simulink model "task_1"  (R2024a)
settings: Solver=VariableStepAuto  StartTime=0.0  StopTime=10.0  RelTol=1e-3
libraries: simulink x1
settings Model: Creator=alexe  LastModifiedBy=alexe

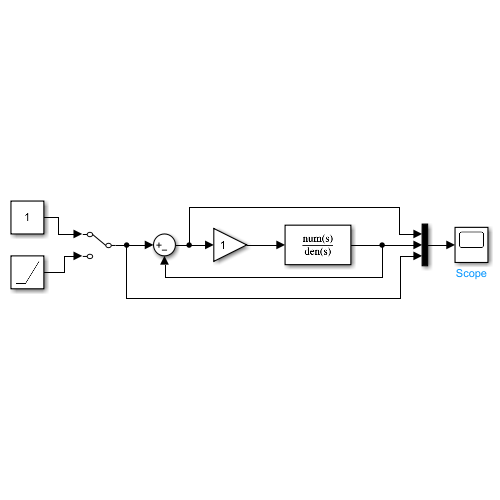
[thumbnail: Simulink's stored preview of the top-level diagram]
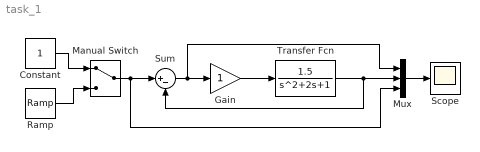
== system task_1 ==
  Constant : Constant
  Gain : Gain
  Manual Switch : ManualSwitch
  Mux : Mux  Inputs=3
  Ramp : simulink/Sources/Ramp  slope=1  start=0  InitialOutput=0
  Scope : Scope
  Sum : Sum  Inputs=|+-
  Transfer Fcn : TransferFcn  Numerator=[1.5]
  wires:
  Constant/1 -> Manual Switch/1
  Ramp/1 -> Manual Switch/2
  Manual Switch/1 -> Mux/3, Sum/1
  Sum/1 -> Mux/1, Gain/1
  Gain/1 -> Transfer Fcn/1
  Transfer Fcn/1 -> Sum/2, Mux/2
  Mux/1 -> Scope/1
